simulink model "urinario_PID"  (R2023a)
settings: Solver=ode15s  StartTime=0.0  StopTime=10.0  MaxStep=1e-3  RelTol=1e-3
libraries: slpidlib x1
settings Model: Creator=najap  LastModifiedBy=najap
settings DataIOCC: ReturnWorkspaceOutputs=off  TimeSaveName=t
settings DebuggingCC: AlgebraicLoopMsg=none  ArtificialAlgebraicLoopMsg=none  MaxConsecutiveZCsMsg=none  ModelReferenceExtraNoncontSigs=none  OperatingPointInterfaceChecksumMismatchMsg=none

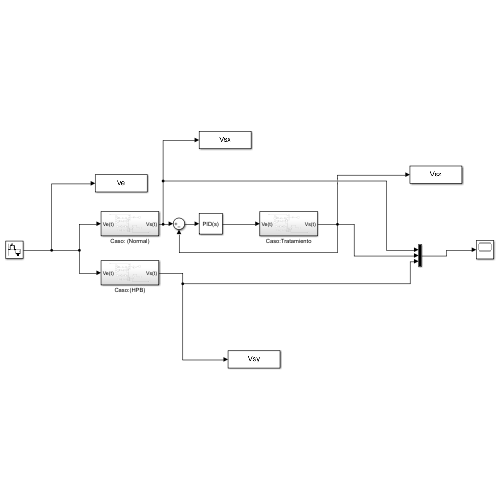
[thumbnail: Simulink's stored preview of the top-level diagram]
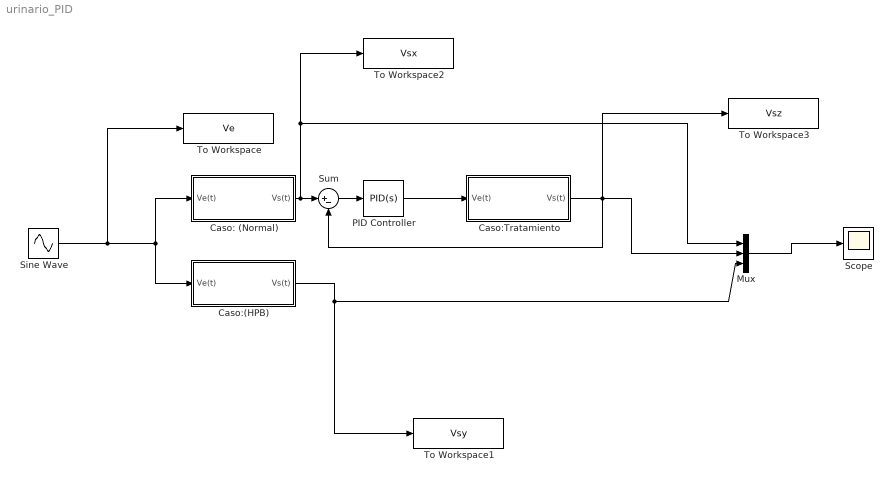
== system urinario_PID ==
  Caso: (Normal) : Subsystem
  Caso:(HPB) : Subsystem
  Caso:Tratamiento : Subsystem
  Mux : Mux  Inputs=3
  PID Controller : slpidlib/PID Controller  Controller=PID  Form=Parallel  TimeDomain=Continuous-time  UseExternalTs=off  SampleTime=-1  IntegratorMethod=Forward Euler  FilterMethod=Forward Euler  ControllerParametersSource=internal  P=37.5678  I=1936.8002  UseKiTs=off  D=1936.8002  N=712.6451  UseFilter=on  TunerSelectOption=Transfer Function Based (PID Tuner App)  InitialConditionSource=internal  InitialConditionForIntegrator=0  InitialConditionForFilter=0  DifferentiatorICPrevScaledInput=0  ExternalReset=none  TrackingMode=off  Kt=1  LimitOutput=off  SatLimitsSource=internal  UpperSaturationLimit=inf  LowerSaturationLimit=-inf  LinearizeAsGain=on  AntiWindupMode=none  Kb=1  LimitIntegrator=off  UpperIntegratorSaturationLimit=inf  LowerIntegratorSaturationLimit=-inf  POutMin=[]  POutMax=[]  IOutMin=[]  IOutMax=[]  DOutMin=[]  DOutMax=[]  NOutMin=[]  NOutMax=[]  SumOutMin=[]  SumOutMax=[]  SaturationOutMin=[]  SaturationOutMax=[]  PParamMin=[]  PParamMax=[]  IParamMin=[]  IParamMax=[]  DParamMin=[]  DParamMax=[]  NParamMin=[]  NParamMax=[]  KbParamMin=[]  KbParamMax=[]  KtParamMin=[]  KtParamMax=[]  KbOutMin=[]  KbOutMax=[]  KtOutMin=[]  KtOutMax=[]  IntegratorOutMin=[]  IntegratorOutMax=[]  FilterOutMin=[]  FilterOutMax=[]  SumI1OutMin=[]  SumI1OutMax=[]  SumI2OutMin=[]  SumI2OutMax=[]  SumI3OutMin=[]  SumI3OutMax=[]  SumI4OutMin=[]  SumI4OutMax=[]  SumDOutMin=[]  SumDOutMax=[]  DifferentiatorOutMin=[]  DifferentiatorOutMax=[]  FilterDiffOutCoefMin=[]  FilterDiffOutCoefMax=[]  ReciprocalOutMin=[]  ReciprocalOutMax=[]  SumDenOutMin=[]  SumDenOutMax=[]  SumNumOutMin=[]  SumNumOutMax=[]  DivideOutMin=[]  DivideOutMax=[]  UdiffTsProdOutMin=[]  UdiffTsProdOutMax=[]  NTsProdOutMin=[]  NTsProdOutMax=[]  UintegralTsProdOutMin=[]  UintegralTsProdOutMax=[]  UngainTsProdOutMin=[]  UngainTsProdOutMax=[]  ClampingZeroOutDataTypeStr=Inherit: Inherit via back propagation  ClampingZeroOutMin=[]  ClampingZeroOutMax=[]  FilterDenConstantOutDataTypeStr=Inherit: Inherit via back propagation  FilterDenConstantOutMin=[]  FilterDenConstantOutMax=[]  PCopyOutDataTypeStr=Inherit: Inherit via back propagation  PCopyOutMin=[]  PCopyOutMax=[]  NCopyOutDataTypeStr=Inherit: Inherit via back propagation  NCopyOutMin=[]  NCopyOutMax=[]  IntegratorContinuousStateAttributes=''  IntegratorStateMustResolveToSignalObject=off  IntegratorRTWStateStorageClass=Auto  FilterContinuousStateAttributes=''  FilterStateMustResolveToSignalObject=off  FilterRTWStateStorageClass=Auto  ParallelPVariant=InternalParameters  IdealPVariant=Disabled  IVariant=InternalParameters  DVariant=InternalParameters  IntegratorVariant=Continuous  SatVariant=Disabled  AWVariant=Passthrough  PCopyVariant=Disabled  TRVariant=Disabled  FdbkBlocksVariant=Forward  IdealPFdbkVariant=Disabled  SatFdbkVariant=Disabled  DerivativeFilterVariant=ContFilter  NVariant=InternalParameters  NCopyVariant=Disabled  FilterICVariant=InternalICsFilter  IntegratorICVariant=InternalICs  ExternalResetVariant=Disabled  TRSumVariant=Passthrough  SumFdbkVariant=Disabled  SumVariant=Sum_PID  TsampFilterVariant=InternalTs  TsampNgainVariant=Passthrough  TsampIntegralVariant=Disabled_SignalSpec  ExternalSaturationOutDataTypeStr=Inherit: Same as second input
  Scope : Scope
  Sine Wave : Sin  Frequency=1.5708  SampleTime=0.001
  Sum : Sum  Inputs=|+-
  To Workspace : ToWorkspace  VariableName=Ve  SaveFormat=Timeseries  SampleTime=-1
  To Workspace1 : ToWorkspace  VariableName=Vsy  SaveFormat=Timeseries  SampleTime=-1
  To Workspace2 : ToWorkspace  VariableName=Vsx  SaveFormat=Timeseries  SampleTime=-1
  To Workspace3 : ToWorkspace  VariableName=Vsz  SaveFormat=Timeseries  SampleTime=-1
  wires:
  Mux/1 -> Scope/1
  Sine Wave/1 -> To Workspace/1, Caso: (Normal)/1(Ve(t)), Caso:(HPB)/1(Ve(t))
  Caso:(HPB)/1(Vs(t)) -> To Workspace1/1, Mux/3
  Caso: (Normal)/1(Vs(t)) -> To Workspace2/1, Mux/1, Sum/1
  Sum/1 -> PID Controller/1
  PID Controller/1 -> Caso:Tratamiento/1(Ve(t))
  Caso:Tratamiento/1(Vs(t)) -> To Workspace3/1, Sum/2, Mux/2

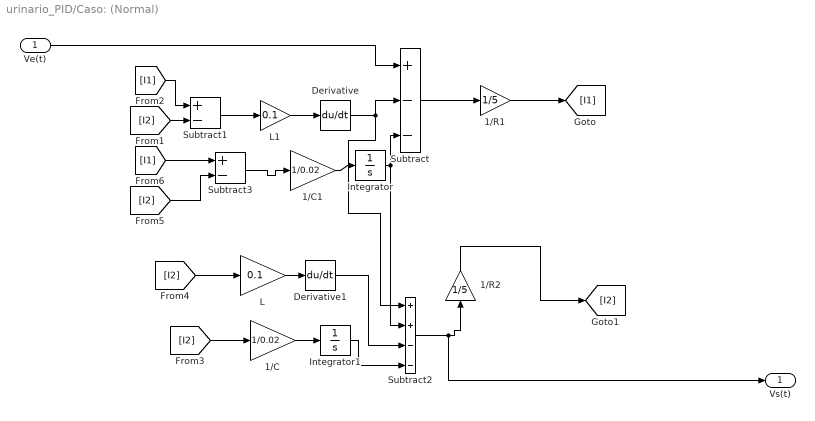
== system urinario_PID/Caso: (Normal) ==
  Ve(t) : Inport
  1/C : Gain  Gain=1/0.02
  1/C1 : Gain  Gain=1/0.02
  1/R1 : Gain  Gain=1/5
  1/R2 : Gain  Gain=1/5
  Derivative : Derivative
  Derivative1 : Derivative
  Integrator : Integrator
  Integrator1 : Integrator
  L : Gain  Gain=0.1
  L1 : Gain  Gain=0.1
  Subtract : Sum  Inputs=+--
  Subtract1 : Sum  Inputs=+-
  Subtract2 : Sum  Inputs=++--
  Subtract3 : Sum  Inputs=+-
  Vs(t) : Outport
  wires:
  [I2] -> L/1
  Ve(t)/1 -> Subtract/1
  Subtract3/1 -> 1/C1/1
  Subtract2/1 -> Vs(t)/1, 1/R2/1
  Subtract1/1 -> L1/1
  [I1] -> Subtract1/1
  [I2] -> Subtract1/2
  [I2] -> Subtract3/2
  [I1] -> Subtract3/1
  1/R2/1 -> [I2]
  Derivative/1 -> Subtract/2, Subtract2/1
  L1/1 -> Derivative/1
  1/C1/1 -> Integrator/1
  Integrator/1 -> Subtract/3, Subtract2/2
  Subtract/1 -> 1/R1/1
  1/R1/1 -> [I1]
  L/1 -> Derivative1/1
  Derivative1/1 -> Subtract2/3
  [I2] -> 1/C/1
  Integrator1/1 -> Subtract2/4
  1/C/1 -> Integrator1/1

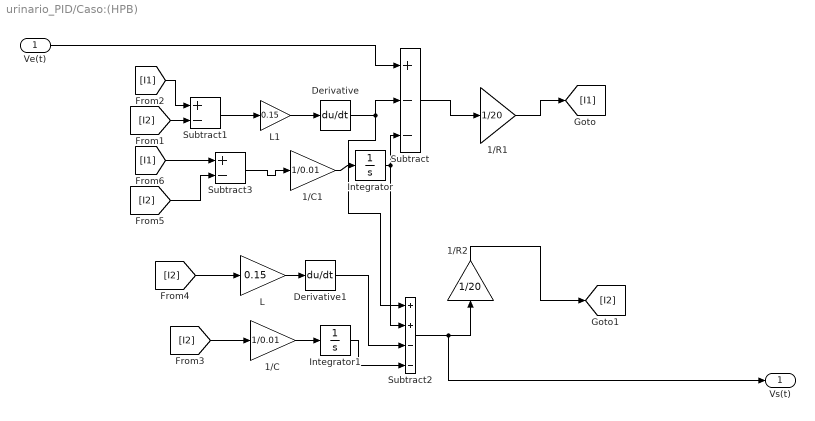
== system urinario_PID/Caso:(HPB) ==
  Ve(t) : Inport
  1/C : Gain  Gain=1/0.01
  1/C1 : Gain  Gain=1/0.01
  1/R1 : Gain  Gain=1/20
  1/R2 : Gain  Gain=1/20
  Derivative : Derivative
  Derivative1 : Derivative
  Integrator : Integrator
  Integrator1 : Integrator
  L : Gain  Gain=0.15
  L1 : Gain  Gain=0.15
  Subtract : Sum  Inputs=+--
  Subtract1 : Sum  Inputs=+-
  Subtract2 : Sum  Inputs=++--
  Subtract3 : Sum  Inputs=+-
  Vs(t) : Outport
  wires:
  L/1 -> Derivative1/1
  Derivative1/1 -> Subtract2/3
  1/C/1 -> Integrator1/1
  Integrator1/1 -> Subtract2/4
  Subtract/1 -> 1/R1/1
  1/R2/1 -> [I2]
  Derivative/1 -> Subtract/2, Subtract2/1
  [I2] -> 1/C/1
  1/C1/1 -> Integrator/1
  1/R1/1 -> [I1]
  L1/1 -> Derivative/1
  [I2] -> L/1
  Integrator/1 -> Subtract/3, Subtract2/2
  Subtract1/1 -> L1/1
  Ve(t)/1 -> Subtract/1
  [I2] -> Subtract1/2
  Subtract3/1 -> 1/C1/1
  Subtract2/1 -> Vs(t)/1, 1/R2/1
  [I1] -> Subtract1/1
  [I2] -> Subtract3/2
  [I1] -> Subtract3/1

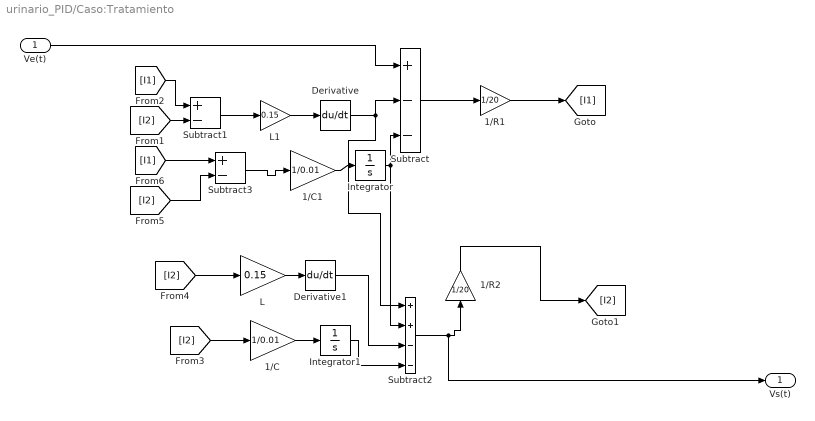
== system urinario_PID/Caso:Tratamiento ==
  Ve(t) : Inport
  1/C : Gain  Gain=1/0.01
  1/C1 : Gain  Gain=1/0.01
  1/R1 : Gain  Gain=1/20
  1/R2 : Gain  Gain=1/20
  Derivative : Derivative
  Derivative1 : Derivative
  Integrator : Integrator
  Integrator1 : Integrator
  L : Gain  Gain=0.15
  L1 : Gain  Gain=0.15
  Subtract : Sum  Inputs=+--
  Subtract1 : Sum  Inputs=+-
  Subtract2 : Sum  Inputs=++--
  Subtract3 : Sum  Inputs=+-
  Vs(t) : Outport
  wires:
  L/1 -> Derivative1/1
  Derivative1/1 -> Subtract2/3
  1/C/1 -> Integrator1/1
  Integrator1/1 -> Subtract2/4
  Subtract/1 -> 1/R1/1
  1/R2/1 -> [I2]
  Derivative/1 -> Subtract/2, Subtract2/1
  [I2] -> 1/C/1
  1/C1/1 -> Integrator/1
  1/R1/1 -> [I1]
  L1/1 -> Derivative/1
  [I2] -> L/1
  Integrator/1 -> Subtract/3, Subtract2/2
  Subtract1/1 -> L1/1
  Ve(t)/1 -> Subtract/1
  [I2] -> Subtract1/2
  Subtract3/1 -> 1/C1/1
  Subtract2/1 -> Vs(t)/1, 1/R2/1
  [I1] -> Subtract1/1
  [I2] -> Subtract3/2
  [I1] -> Subtract3/1
